simulink model "Emergency smart breaking-Fuzzy"  (R2019b)
settings: Solver=ode45  StartTime=0.0  StopTime=100  MaxStep=1e-2  MinStep=1e-5  RelTol=1e-6
model workspace (MAT data in the model file):
  Ainit = 3
values from neighbouring files (symbols this model uses):
  Dist_init = 100    [Emergency smart breaking-FUZZY_init.m]
  maxdistp = 25    [Emergency smart breaking-FUZZY_init.m]
  maxspeeds = maxspeeds_kmh/3.6    (= 11.1111111111)    [Emergency smart breaking-FUZZY_init.m]
  mean_dist = 35    [Emergency smart breaking-FUZZY_init.m]
  mean_speed = mean_speed_kmh/3.6    (= 11.9444444444)    [Emergency smart breaking-FUZZY_init.m]
  mindistL = 40    [Emergency smart breaking-FUZZY_init.m]
  minspeedf = minspeedf_kmh/3.6    (= 14.4444444444)    [Emergency smart breaking-FUZZY_init.m]
  sigma_dist = 2    [Emergency smart breaking-FUZZY_init.m]
  sigma_speed = sigma_speed_kmh/3.6    (= 0.833333333333)    [Emergency smart breaking-FUZZY_init.m]
  Vinit = Vinit_kmh/3.6    (= 25)    [Emergency smart breaking-FUZZY_init.m]
settings Model: Creator=Alexis  LastModifiedBy=ravisanjai
settings SolverCC: ShapePreserveControl=EnableAll  ZeroCrossControl=EnableAll  ZeroCrossAlgorithm=Adaptive
settings DataIOCC: ReturnWorkspaceOutputs=off
settings DebuggingCC: ArithmeticOperatorsInVariantConditions=warning
settings SFSimCC: SimUseLocalCustomCode=off  CustomCodeUndefinedFunction=UseInterfaceOnly
settings RTWCC: RTWUseLocalCustomCode=off
settings CodeAppCC: StateflowObjectComments=on

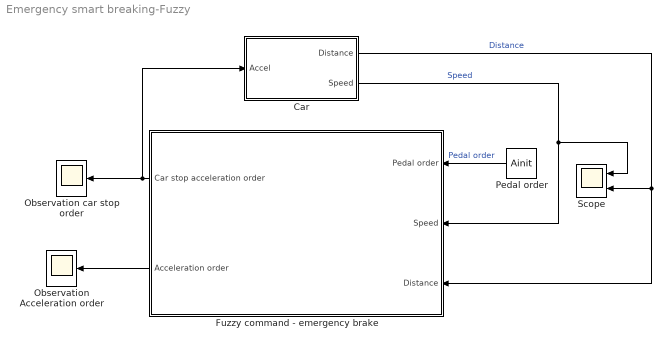
== system Emergency smart breaking-Fuzzy ==
  Car : Subsystem
  Fuzzy command - emergency brake : Subsystem
  Observation Acceleration order : Scope
  Observation car stop order : Scope
  Pedal order : Constant  Value=Ainit
  Scope : Scope  NumInputPorts=2
  wires:
  Car/1(Distance) -> Scope/2, Fuzzy command - emergency brake/3(Distance)  "Distance"
  Car/2(Speed) -> Scope/1, Fuzzy command - emergency brake/2(Speed)  "Speed"
  Fuzzy command - emergency brake/2(Acceleration order) -> Observation Acceleration order/1
  Pedal order/1 -> Fuzzy command - emergency brake/1(Pedal order)  "Pedal order"
  Fuzzy command - emergency brake/1(Car stop acceleration order) -> Car/1(Accel), Observation car stop order/1

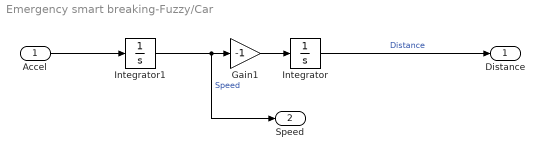
== system Emergency smart breaking-Fuzzy/Car ==
  Accel : Inport
  Gain1 : Gain  Gain=-1
  Integrator : Integrator  InitialCondition=Dist_init  LimitOutput=on  LowerSaturationLimit=0
  Integrator1 : Integrator  InitialCondition=Vinit  LowerSaturationLimit=0
  Distance : Outport
  Speed : Outport  Port=2
  wires:
  Integrator/1 -> Distance/1  "Distance"
  Accel/1 -> Integrator1/1
  Integrator1/1 -> Speed/1, Gain1/1  "Speed"
  Gain1/1 -> Integrator/1

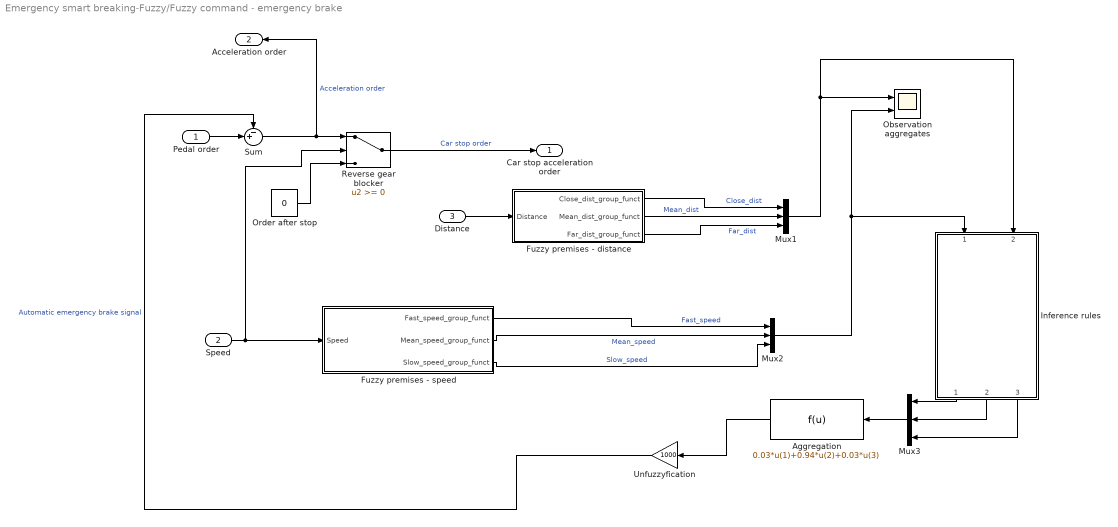
== system Emergency smart breaking-Fuzzy/Fuzzy command - emergency brake ==
  Pedal order : Inport
  Speed : Inport  Port=2
  Distance : Inport  Port=3
  Aggregation : Fcn  Expr=0.03*u(1)+0.94*u(2)+0.03*u(3)
  Fuzzy premises - distance : Subsystem
  Fuzzy premises - speed : Subsystem
  Inference rules : Subsystem
  Mux1 : Mux  Inputs=3
  Mux2 : Mux  Inputs=3
  Mux3 : Mux  Inputs=3
  Observation aggregates : Scope  NumInputPorts=2
  Order after stop : Constant  Value=0
  Reverse gear blocker : Switch
  Sum : Sum  Inputs=-+|
  Unfuzzyfication : Gain  Gain=1000
  Car stop acceleration order : Outport
  Acceleration order : Outport  Port=2
  wires:
  Inference rules/1(Emergency) -> Mux3/1
  Fuzzy premises - speed/2(Mean_speed_group_funct) -> Mux2/2  "Mean_speed"
  Fuzzy premises - distance/2(Mean_dist_group_funct) -> Mux1/2  "Mean_dist"
  Mux2/1 -> Inference rules/1(Speed_group_funct), Observation aggregates/2
  Speed/1 -> Reverse gear blocker/2, Fuzzy premises - speed/1(Speed)
  Distance/1 -> Fuzzy premises - distance/1(Distance)
  Mux1/1 -> Inference rules/2(Dist_group_funct), Observation aggregates/1
  Fuzzy premises - distance/1(Close_dist_group_funct) -> Mux1/1  "Close_dist"
  Aggregation/1 -> Unfuzzyfication/1
  Order after stop/1 -> Reverse gear blocker/3
  Inference rules/2(Warning 1) -> Mux3/2
  Mux3/1 -> Aggregation/1
  Inference rules/3(Warning 2) -> Mux3/3
  Fuzzy premises - speed/3(Slow_speed_group_funct) -> Mux2/3  "Slow_speed"
  Fuzzy premises - speed/1(Fast_speed_group_funct) -> Mux2/1  "Fast_speed"
  Fuzzy premises - distance/3(Far_dist_group_funct) -> Mux1/3  "Far_dist"
  Pedal order/1 -> Sum/2
  Unfuzzyfication/1 -> Sum/1  "Automatic emergency brake signal"
  Reverse gear blocker/1 -> Car stop acceleration order/1  "Car stop order"
  Sum/1 -> Acceleration order/1, Reverse gear blocker/1  "Acceleration order"

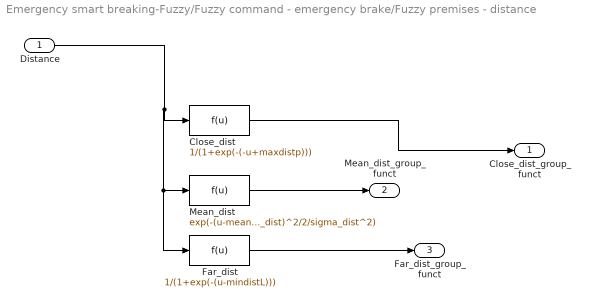
== system Emergency smart breaking-Fuzzy/Fuzzy command - emergency brake/Fuzzy premises - distance ==
  Distance : Inport
  Close_dist : Fcn  Expr=1/(1+exp(-(-u+maxdistp)))
  Far_dist : Fcn  Expr=1/(1+exp(-(u-mindistL)))
  Mean_dist : Fcn  Expr=exp(-(u-mean_dist)^2/2/sigma_dist^2)
  Close_dist_group_funct : Outport
  Mean_dist_group_funct : Outport  Port=2
  Far_dist_group_funct : Outport  Port=3
  wires:
  Far_dist/1 -> Far_dist_group_funct/1
  Close_dist/1 -> Close_dist_group_funct/1
  Distance/1 -> Far_dist/1, Mean_dist/1, Close_dist/1
  Mean_dist/1 -> Mean_dist_group_funct/1

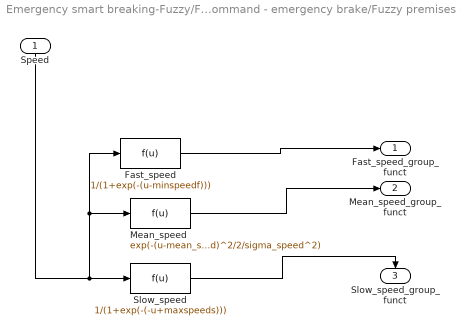
== system Emergency smart breaking-Fuzzy/Fuzzy command - emergency brake/Fuzzy premises - speed ==
  Speed : Inport
  Fast_speed : Fcn  Expr=1/(1+exp(-(u-minspeedf)))
  Mean_speed : Fcn  Expr=exp(-(u-mean_speed)^2/2/sigma_speed^2)
  Slow_speed : Fcn  Expr=1/(1+exp(-(-u+maxspeeds)))
  Fast_speed_group_funct : Outport
  Mean_speed_group_funct : Outport  Port=2
  Slow_speed_group_funct : Outport  Port=3
  wires:
  Slow_speed/1 -> Slow_speed_group_funct/1
  Fast_speed/1 -> Fast_speed_group_funct/1
  Speed/1 -> Slow_speed/1, Fast_speed/1, Mean_speed/1
  Mean_speed/1 -> Mean_speed_group_funct/1

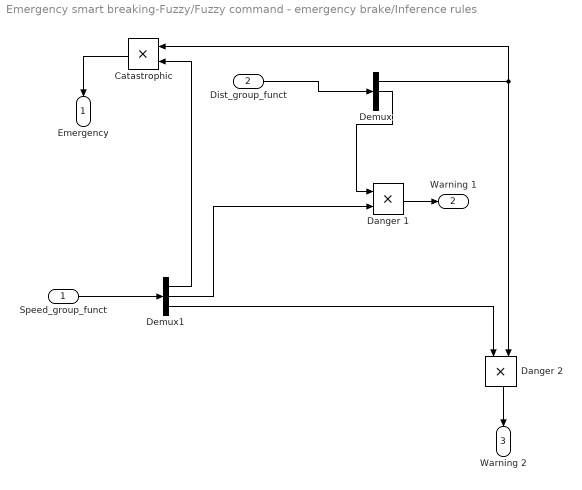
== system Emergency smart breaking-Fuzzy/Fuzzy command - emergency brake/Inference rules ==
  Speed_group_funct : Inport
  Dist_group_funct : Inport  Port=2
  Catastrophic : Product
  Danger 1 : Product
  Danger 2 : Product
  Demux : Demux  Outputs=3
  Demux1 : Demux  Outputs=3
  Emergency : Outport
  Warning 1 : Outport  Port=2
  Warning 2 : Outport  Port=3
  wires:
  Danger 1/1 -> Warning 1/1
  Danger 2/1 -> Warning 2/1
  Catastrophic/1 -> Emergency/1
  Demux/2 -> Danger 1/1
  Demux1/3 -> Danger 2/1
  Demux1/2 -> Danger 1/2
  Demux1/1 -> Catastrophic/2
  Demux/1 -> Danger 2/2, Catastrophic/1
  Dist_group_funct/1 -> Demux/1
  Speed_group_funct/1 -> Demux1/1
